simulink model "QCar2_hardware_test_rp_lidar_a2"  (R2023a)
settings: Solver=ode2  StartTime=0.0  StopTime=inf  FixedStep=0.1  RelTol=1e-3  EnableMultiTasking=on
undefined symbols (not defined in the file): Point
libraries: quarc_library x4
settings Model: SimulationMode=external  ExtModeTrigDuration=10000  Creator=Quanser  LastModifiedBy=Lorena Gonzalez
settings SolverCC: AlgebraicLoopSolver=TrustRegion  PositivePriorityOrder=on
settings DataIOCC: ReturnWorkspaceOutputs=off
settings DebuggingCC: UnconnectedInputMsg=warning  UnconnectedOutputMsg=warning  UnconnectedLineMsg=warning  ArithmeticOperatorsInVariantConditions=warning
settings HardwareCC: ProdBitPerLong=64  ProdLargestAtomicInteger=LongLong  ProdLargestAtomicFloat=Double  ProdLongLongMode=on  ProdHWDeviceType=ARM Compatible->ARM 64-bit (LP64)
settings ModelReferenceCC: EnableRefExpFcnMdlSchedulingChecks=on
settings SFSimCC: CustomCodeUndefinedFunction=UseInterfaceOnly
settings RTWCC: Description=QUARC Linux QCar2 Target Using Toolchain  SystemTargetFile=quarc_linux_qcar2.tlc  TemplateMakefile=quarc_default_tmf  Toolchain=QUARC linux_qcar2 | gmake (64-bit Windows)  BuildConfiguration=Faster Runs
settings STFCustomTargetCC: SystemTargetFile=quarc_linux_qcar2.tlc
settings GRTTargetCC: ParMdlRefBuildCompliant=off  CompOptLevelCompliant=off  CombineOutputUpdateFcns=off  MatFileLogging=off  CPPClassGenCompliant=off  GRTInterface=on  ExtMode=on  ExtModeMexFile=quarc_comm  ExtModeMexArgs='-w -d /tmp -uri %u','tcpip://192.168.3.23:17001'

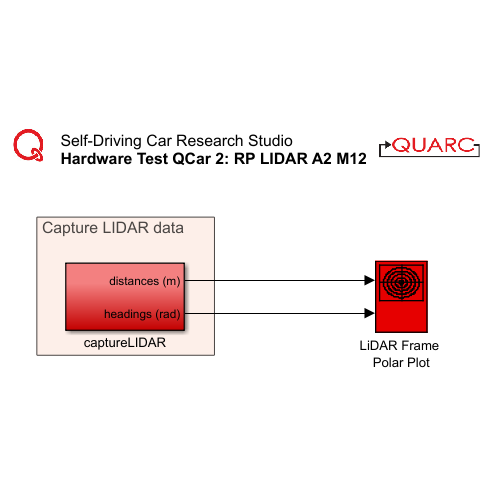
[thumbnail: Simulink's stored preview of the top-level diagram]
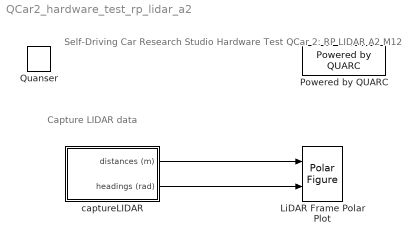
== system QCar2_hardware_test_rp_lidar_a2 ==
  note: Capture LIDAR data
  note: Self-Driving Car Research Studio
      | Hardware Test QCar 2: RP LIDAR A2 M12
  LiDAR Frame Polar Plot : quarc_library/Sinks/Figures/Polar Figure  figure_mode=Use figure window  figure_tag=figure1  axes_tag=axes1  plot_mode=Frame-based  minimum_rho=0  maximum_rho=5  minimum_theta=0  maximum_theta=360  zero_location=left  direction=clockwise  buffer_size=1000  update_rate=1  sample_time=-1  initial_position="485.8         257.8         653.6         474.4"  initial_visibility=on  line1_style=None  line1_width=1  line1_color=[0 0 0]  marker1=Point (.)  marker1_size=1  marker1_edge_color=[0 0.447059 0.741176]  marker1_face_color=[0 0.447059 0.741176]  line2_style=Solid line (-)  line2_width=0.5  line2_color=[0.85098 0.32549 0.0980392]  marker2=None  marker2_size=6  marker2_edge_color=[0.85098 0.32549 0.0980392]  marker2_face_color=[0.85098 0.32549 0.0980392]  line3_style=Solid line (-)  line3_width=0.5  line3_color=[0.929412 0.694118 0.12549]  marker3=None  marker3_size=6  marker3_edge_color=[0.929412 0.694118 0.12549]  marker3_face_color=[0.929412 0.694118 0.12549]  line4_style=Solid line (-)  line4_width=0.5  line4_color=[0.494118 0.184314 0.556863]  marker4=None  marker4_size=6  marker4_edge_color=[0.494118 0.184314 0.556863]  marker4_face_color=[0.494118 0.184314 0.556863]  line5_style=Solid line (-)  line5_width=0.5  line5_color=[0.466667 0.67451 0.188235]  marker5=None  marker5_size=6  marker5_edge_color=[0.466667 0.67451 0.188235]  marker5_face_color=[0.466667 0.67451 0.188235]
      settings: SourceProductName=QUARC Targets
  Powered by QUARC : quarc_library/Logos/Powered by QUARC
  Quanser : quarc_library/Logos/Quanser
  captureLIDAR : Subsystem
  wires:
  captureLIDAR/1(distances (m)) -> LiDAR Frame Polar Plot/1
  captureLIDAR/2(headings (rad)) -> LiDAR Frame Polar Plot/2

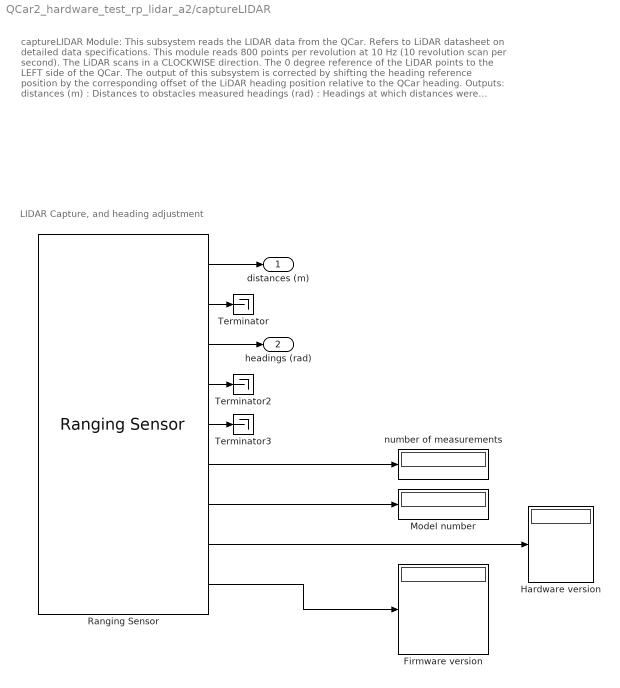
== system QCar2_hardware_test_rp_lidar_a2/captureLIDAR ==
  note: LIDAR Capture, and heading adjustment
  note: captureLIDAR Module:
      |
      | This subsystem reads the LIDAR data from the QCar. Refers to LiDAR datasheet on detailed data specifications.
      | This module reads 800 points per revolution at 10 Hz (10 revolution scan per second).
      | The LiDAR scans in a CLOCKWISE direction. The 0 degree reference of the LiDAR points to the LEFT side of the QCar.
      | The output of this subsystem is corrected by shifting the heading reference position by the corresponding offset of the LiDAR heading position relative to the QCar heading.
      |
      | Outputs:
      | distances (m) : Distances to obstacles measured
      | headings (rad) : Headings at which distances were measured (corrected relative to QCar heading)
  Firmware version : Display
  Hardware version : Display
  Model number : Display
  Ranging Sensor : quarc_library/Devices/Third-Party/Sensors/Ranging Sensor  sensor_type=RPLidar LIDAR  uri=serial-cpu://localhost:1?baud='256000',word='8',parity='none',stop='1',flow='none',dsr='on'  ranging_distance=Long  timing_budget=0.033  measurement_period=0.0005  output_mode=Fixed-size output  samples_per_revolution=1000  max_distance=0.050  max_angle=5  sample_time=qc_get_step_size  show_versions=on  active=on
      settings: SourceProductName=QUARC Targets
  Terminator : Terminator
  Terminator2 : Terminator
  Terminator3 : Terminator
  number of measurements : Display
  distances (m) : Outport  VectorParamsAs1DForOutWhenUnconnected=off
  headings (rad) : Outport  Port=2  VectorParamsAs1DForOutWhenUnconnected=off
  wires:
  Ranging Sensor/2 -> Terminator/1
  Ranging Sensor/4 -> Terminator2/1
  Ranging Sensor/5 -> Terminator3/1
  Ranging Sensor/1 -> distances (m)/1
  Ranging Sensor/6 -> number of measurements/1
  Ranging Sensor/3 -> headings (rad)/1
  Ranging Sensor/7 -> Model number/1
  Ranging Sensor/8 -> Hardware version/1
  Ranging Sensor/9 -> Firmware version/1
